simulink subsystem "Inverter_and_Motor"  (R2024b)
settings: Solver=VariableStepAuto  StartTime=0.0  StopTime=10.0  RelTol=1e-3
values from neighbouring files (symbols this model uses):
  PI_params = mcb.internal.SetControllerParameters(pmsm,inverter,SI_System,T_pwm,Ts,Ts_speed)    [mchp_pmsm_foc_encoder_dsPIC33A_data.m]
  Ts = T_pwm    (= 5e-05)    [mchp_pmsm_foc_encoder_dsPIC33A_data.m]
undefined symbols (not defined in the file or in its folder): inverter, pmsm
libraries: mcbplantlib x1, mcbcontrolslib x1, autolibpmsmexterior x1
settings Model: Creator=I50990  LastModifiedBy=I52209
settings RTWCC: GPUComputeCapability=3.5

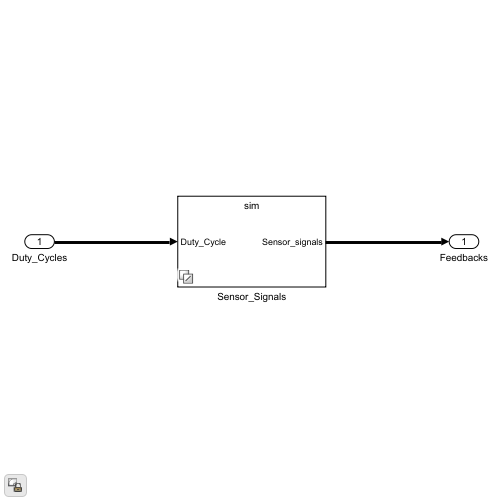
[thumbnail: Simulink's stored preview of the top-level diagram]
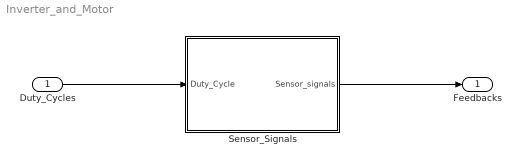
== system Inverter_and_Motor ==
  Duty_Cycles : Inport
  Sensor_Signals : Subsystem  Variant=on  VariantControlMode=sim codegen switching
  Feedbacks : Outport  VectorParamsAs1DForOutWhenUnconnected=off
  wires:
  Sensor_Signals/1(Sensor_signals) -> Feedbacks/1
  Duty_Cycles/1 -> Sensor_Signals/1(Duty_Cycle)

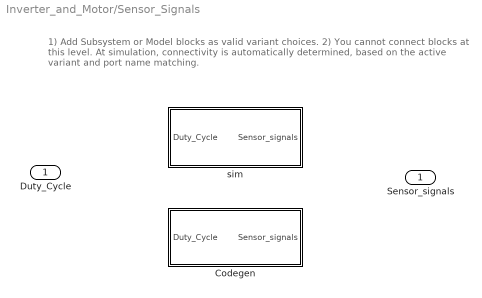
== system Inverter_and_Motor/Sensor_Signals ==
  note: 1) Add Subsystem or Model blocks as valid variant choices.
      | 2) You cannot connect blocks at this level. At simulation, connectivity is automatically
      | determined, based on the active variant and port name matching.
  Duty_Cycle : Inport
  Codegen : Subsystem  VariantControl=(codegen)
  sim : Subsystem  VariantControl=(sim)
  Sensor_signals : Outport

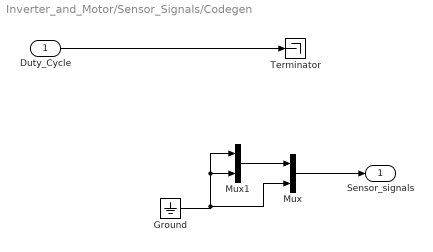
== system Inverter_and_Motor/Sensor_Signals/Codegen ==
  Duty_Cycle : Inport
  Ground : Ground
  Mux : Mux  Inputs=2
  Mux1 : Mux  Inputs=2
  Terminator : Terminator
  Sensor_signals : Outport
  wires:
  Ground/1 -> Mux/2, Mux1/1, Mux1/2
  Mux1/1 -> Mux/1
  Mux/1 -> Sensor_signals/1
  Duty_Cycle/1 -> Terminator/1

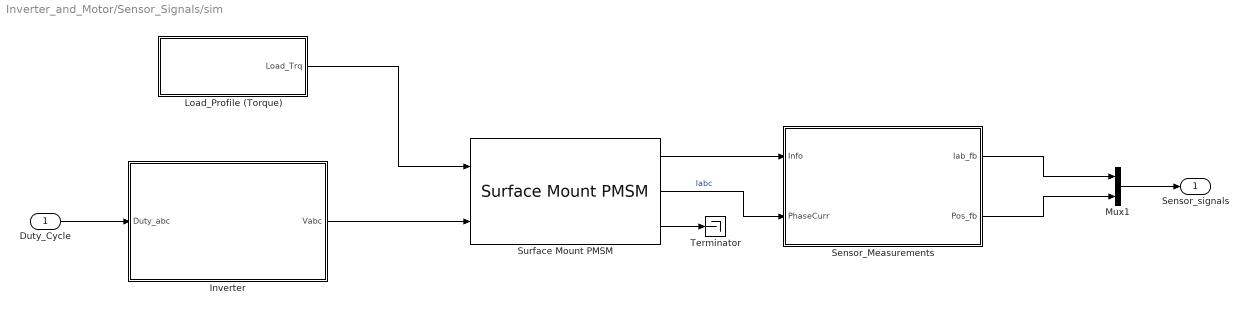
== system Inverter_and_Motor/Sensor_Signals/sim ==
  Duty_Cycle : Inport
  Inverter : Subsystem
  Load_Profile (Torque) : Subsystem
  Mux1 : Mux  Inputs=2
  Sensor_Measurements : Subsystem
  Surface Mount PMSM : autolibpmsmexterior/Surface Mount PMSM  port_config=Torque  sim_type=Discrete  Ts=Ts  P=pmsm.p  Rs=pmsm.Rs  Ldq_=pmsm.Ld  KConstText=Back-emf constant (Ke):  lambda_pm=0.2205  Ke=pmsm.Ke  Kt=1.323  mechanical=[pmsm.J, pmsm.B, 0]  idq0=[0 0]  theta_init=0  omega_init=0  KConst=0.2205  lambda_pm_calc=0.0080963  RefBlkName='autolibpmsmexterior/Surface Mount PMSM'  aMode=5  Ldq="[0.0017      0.0017]"
  Terminator : Terminator
  Sensor_signals : Outport
  wires:
  Mux1/1 -> Sensor_signals/1
  Duty_Cycle/1 -> Inverter/1(Duty_abc)
  Load_Profile (Torque)/1(Load_Trq) -> Surface Mount PMSM/1
  Surface Mount PMSM/1 -> Sensor_Measurements/1(Info)
  Surface Mount PMSM/2 -> Sensor_Measurements/2(PhaseCurr)  "Iabc"
  Sensor_Measurements/2(Pos_fb) -> Mux1/2
  Inverter/1(Vabc) -> Surface Mount PMSM/2
  Sensor_Measurements/1(Iab_fb) -> Mux1/1
  Surface Mount PMSM/3 -> Terminator/1

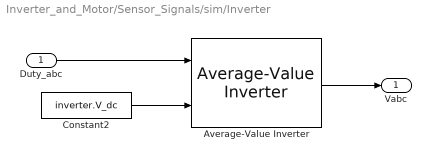
== system Inverter_and_Motor/Sensor_Signals/sim/Inverter ==
  Duty_abc : Inport
  Average-Value Inverter : mcbplantlib/Average-Value Inverter
  Constant2 : Constant  Value=inverter.V_dc  OutDataTypeStr=single  SampleTime=-1
  Vabc : Outport  VectorParamsAs1DForOutWhenUnconnected=off
  wires:
  Constant2/1 -> Average-Value Inverter/2
  Duty_abc/1 -> Average-Value Inverter/1
  Average-Value Inverter/1 -> Vabc/1

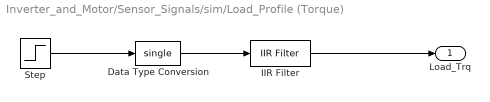
== system Inverter_and_Motor/Sensor_Signals/sim/Load_Profile (Torque) ==
  Data Type Conversion : DataTypeConversion  OutDataTypeStr=single  SaturateOnIntegerOverflow=off  RndMeth=Floor
  IIR Filter : mcbcontrolslib/IIR Filter  VariantControl=Low Pass Filter  VariantSelect=Low-pass  FilterConstantInputType=Specify via dialog  Filter_constant=0.01  advancedSettings=off  Ts=50e-6  cutOff_freq=32.1525
  Step : Step  Time=9  Before=0.01 * pmsm.T_rated  After=0.1 * pmsm.T_rated
  Load_Trq : Outport  VectorParamsAs1DForOutWhenUnconnected=off
  wires:
  Step/1 -> Data Type Conversion/1
  Data Type Conversion/1 -> IIR Filter/1
  IIR Filter/1 -> Load_Trq/1

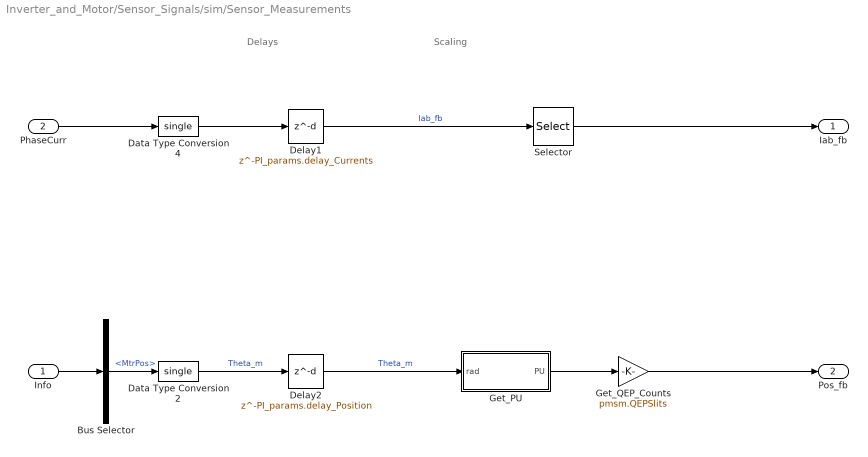
== system Inverter_and_Motor/Sensor_Signals/sim/Sensor_Measurements ==
  note: Scaling
  note: Delays
  Info : Inport
  PhaseCurr : Inport  Port=2
  Bus Selector : BusSelector  OutputSignals=MtrPos
  Data Type Conversion2 : DataTypeConversion  OutDataTypeStr=single  RndMeth=Simplest  SaturateOnIntegerOverflow=off
  Data Type Conversion4 : DataTypeConversion  OutDataTypeStr=single  RndMeth=Simplest  SaturateOnIntegerOverflow=off
  Delay1 : Delay  DelayLength=PI_params.delay_Currents
  Delay2 : Delay  DelayLength=PI_params.delay_Position
  "Get_PU " : Subsystem
  Get_QEP_Counts : Gain  Gain=pmsm.QEPSlits  OutDataTypeStr=single  RndMeth=Simplest
  Selector : Selector  InputPortWidth=3  IndexOptions=Index vector (dialog)  Indices=[1 2]  OutputSizes=1
  Iab_fb : Outport  VectorParamsAs1DForOutWhenUnconnected=off
  Pos_fb : Outport  Port=2  VectorParamsAs1DForOutWhenUnconnected=off
  wires:
  Get_QEP_Counts/1 -> Pos_fb/1
  Selector/1 -> Iab_fb/1
  "Get_PU "/1(PU) -> Get_QEP_Counts/1
  Delay1/1 -> Selector/1  "Iab_fb"
  Data Type Conversion4/1 -> Delay1/1
  PhaseCurr/1 -> Data Type Conversion4/1
  Info/1 -> Bus Selector/1
  Bus Selector/1 -> Data Type Conversion2/1  "<MtrPos>"
  Data Type Conversion2/1 -> Delay2/1  "Theta_m"
  Delay2/1 -> "Get_PU "/1(rad)  "Theta_m"

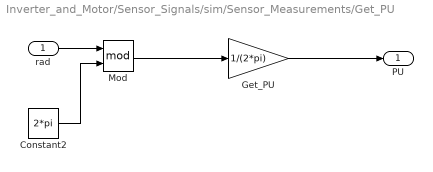
== system Inverter_and_Motor/Sensor_Signals/sim/Sensor_Measurements/Get_PU  ==
  rad : Inport
  Constant2 : Constant  Value=2*pi  OutDataTypeStr=single  SampleTime=-1
  Get_PU : Gain  Gain=1/(2*pi)  OutDataTypeStr=dataType  RndMeth=Simplest
  Mod : Math  Operator=mod
  PU : Outport  VectorParamsAs1DForOutWhenUnconnected=off
  wires:
  Get_PU/1 -> PU/1
  rad/1 -> Mod/1
  Constant2/1 -> Mod/2
  Mod/1 -> Get_PU/1
